simulink model "Assembly"  (R2022b)
settings: Solver=daessc  StartTime=0.0  StopTime=20  MaxStep=1e-3  RelTol=1e-3  AbsTol=1e-3
PreLoadFcn:
  | load environment.mat;
values from neighbouring files (symbols this model uses):
  K_dqdp = 1000    [allData.mat]
  robot =     [allData.mat]
  smoother_length = 4    [allData.mat]
  ts = 0.01    [allData.mat]
undefined symbols (not defined in the file or in its folder): X, Y, Z
libraries: sm_lib x37, nesl_utility x26, dspfactors x8, robotmaniplib x8, simulink x1, dspinverses x1
(part 2 of 2)

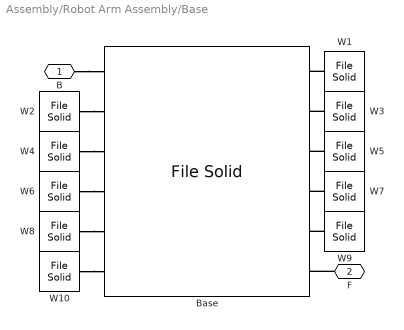
== system Assembly/Robot Arm Assembly/Base ==
  Base : sm_lib/Body Elements/File Solid  ExtGeomFileName=Base.step  UnitType=FromFile  ExtGeomFileUnits=m  StepReaderType=HEX  ExportConvexHullGeometry=off  InertiaType=CalculateFromGeometry  Mass=robot.Solid(19).mass  MassUnits=kg  CenterOfMass=robot.Solid(19).CoM  CenterOfMassUnits=mm  MomentsOfInertia=robot.Solid(19).MoI  MomentsOfInertiaUnits=kg*mm^2  ProductsOfInertia=robot.Solid(19).PoI  ProductsOfInertiaUnits=kg*mm^2  BasedOnType=Density  Density=1000  DensityUnits=kg/m^3  DoExposeReferenceFrame=off  SerializedFrames=<Frames><Frame><Id>Frame1</Id><Value><Name>Origin</Name><Origin><Source>GeometricFeature</Source><FeatureName>segment 442</FeatureName></Origin><PrimaryAxis><DefinedDirection>+Z</DefinedDirection><Source>ReferenceFrame</Source><SourceDirection>-X</SourceDirection><FeatureName></FeatureName></PrimaryAxis><SecondaryAxis><DefinedDirection>+Y</DefinedDirection><Source>ReferenceFrame</Source><SourceDirection>-Y</SourceDirection><FeatureName></FeatureName></SecondaryAxis></Value></Frame><Frame><Id>Frame2</Id><Value><Name>W1</Name><Origin><Source>GeometricFeature</Source><FeatureName>circular curve 177</FeatureName></Origin><PrimaryAxis><DefinedDirection>+Z</DefinedDirection><Source>ReferenceFrame</Source><SourceDirection>+Z</SourceDirection><FeatureName></FeatureName></PrimaryAxis><SecondaryAxis><DefinedDirection>+X</DefinedDirection><Source>ReferenceFrame</Source><SourceDirection>+X</SourceDirection><FeatureName></FeatureName></SecondaryAxis></Value></Frame><Frame><Id>Frame3</Id><Value><Name>W2</Name><Origin><Source>GeometricFeature</Source><FeatureName>circular curve 171</FeatureName></Origin><PrimaryAxis><DefinedDirection>+Z</DefinedDirection><Source>ReferenceFrame</Source><SourceDirection>+Z</SourceDirection><FeatureName></FeatureName></PrimaryAxis><SecondaryAxis><DefinedDirection>+X</DefinedDirection><Source>ReferenceFrame</Source><SourceDirection>+X</SourceDirection><FeatureName></FeatureName></SecondaryAxis></Value></Frame><Frame><Id>Frame4</Id><Value><Name>W3</Name><Origin><Source>GeometricFeature</Source><FeatureName>circular curve 168</FeatureName></Origin><PrimaryAxis><DefinedDirection>+Z</DefinedDirection><Source>ReferenceFrame</Source><SourceDirection>+Z</SourceDirection><FeatureName></FeatureName></PrimaryAxis><SecondaryAxis><DefinedDirection>+X</DefinedDirection><Source>ReferenceFrame</Source><SourceDirection>+X</SourceDirection><FeatureName></FeatureName></SecondaryAxis></Value></Frame><Frame><Id>Frame5</Id><Value><Name>W4</Name><Origin><Source>GeometricFeature</Source><FeatureName>circular curve 174</FeatureName></Origin><PrimaryAxis><DefinedDirection>+Z</DefinedDirection><Source>ReferenceFrame</Source><SourceDirection>+Z</SourceDirection><FeatureName></FeatureName></PrimaryAxis><SecondaryAxis><DefinedDirection>+X</DefinedDirection><Source>ReferenceFrame</Source><SourceDirection>+X</SourceDirection><FeatureName></FeatureName></SecondaryAxis></Value></Frame><Frame><Id>Frame6</Id><Value><Name>W5</Name><Origin><Source>GeometricFeature</Source><FeatureName>circular curve 179</FeatureName></Origin><PrimaryAxis><DefinedDirection>+Z</DefinedDirection><Source>ReferenceFrame</Source><SourceDirection>+Z</SourceDirection><FeatureName></FeatureName></PrimaryAxis><SecondaryAxis><DefinedDirection>+X</DefinedDirection><Source>ReferenceFrame</Source><SourceDirection>+X</SourceDirection><FeatureName></FeatureName></SecondaryAxis></Value></Frame><Frame><Id>Frame7</Id><Value><Name>W6</Name><Origin><Source>GeometricFeature</Source><FeatureName>circular curve 165</FeatureName></Origin><PrimaryAxis><DefinedDirection>+Z</DefinedDirection><Source>ReferenceFrame</Source><SourceDirection>+Z</SourceDirection><FeatureName></FeatureName></PrimaryAxis><SecondaryAxis><DefinedDirection>+X</DefinedDirection><Source>ReferenceFrame</Source><SourceDirection>+X</SourceDirection><FeatureName></FeatureName></SecondaryAxis></Value></Frame><Frame><Id>Frame8</Id><Value><Name>W7</Name><Origin><Source>GeometricFeature</Source><FeatureName>circular curve 157</FeatureName></Origin><PrimaryAxis><DefinedDirection>+Z</DefinedDirection><Source>ReferenceFrame</Source><SourceDirection>+Z</SourceDirection><FeatureName></FeatureName></PrimaryAxis><SecondaryAxis><DefinedDirection>+X</DefinedDirection><Source>ReferenceFrame</Source><SourceDirection>+X</SourceDirection><FeatureName></FeatureName></SecondaryAxis></Value></Frame><Frame><Id>Frame9</Id><Value><Name>W8</Name><Origin><Source>GeometricFeature</Source><FeatureName>circular curve 149</FeatureName></Origin><PrimaryAxis><DefinedDirection>+Z</DefinedDirection><Source>ReferenceFrame</Source><SourceDirection>+Z</SourceDirection><FeatureName></FeatureName></PrimaryAxis><SecondaryAxis><DefinedDirection>+X</DefinedDirection><Source>ReferenceFrame</Source><SourceDirection>+X</SourceDirection><FeatureName></FeatureName></SecondaryAxis></Value></Frame><Frame><Id>Frame10</Id><Value><Name>W9</Name><Origin><Source>GeometricFeature</Source><FeatureName>circular curve 153</FeatureName></Origin><PrimaryAxis><DefinedDirection>+Z</DefinedDirection><Source>ReferenceFrame</Source><SourceDirection>+Z</SourceDirection><FeatureName></FeatureName></PrimaryAxis><SecondaryAxis><DefinedDirection>+X</DefinedDirection><Source>ReferenceFrame</Source><SourceDirection>+X</SourceDirection><FeatureName></FeatureName></SecondaryAxis></Value></Frame><Frame><Id>Frame11</Id><Value><Name>W10</Name><Origin><Source>GeometricFeature</Source><FeatureName>circular curve 161</FeatureName></Origin><PrimaryAxis><DefinedDirection>+Z</DefinedDirection><Source>ReferenceFrame</Source><SourceDirection>+Z</SourceDirection><FeatureName></FeatureName></PrimaryAxis><SecondaryAxis><DefinedDirection>+X</DefinedDirection><Source>ReferenceFrame</Source><SourceDirection>+X</SourceDirection><FeatureName></FeatureName></SecondaryAxis></Value></Frame><Frame><Id>Frame12</Id><Value><Name>F</Name><Origin><Source>GeometricFeature</Source><FeatureName>planar surface 2</FeatureName></Origin><PrimaryAxis><DefinedDirection>+Z</DefinedDirection><Source>ReferenceFrame</Source><SourceDirection>+Z</SourceDirection><FeatureName></FeatureName></PrimaryAxis><SecondaryAxis><DefinedDirection>+X</DefinedDirection><Source>ReferenceFrame</Source><SourceDirection>+X</SourceDirection><FeatureName></FeatureName></SecondaryAxis></Value></Frame></Frames>  GraphicType=FromGeometry  MarkerShape=Sphere  MarkerSize=10  GraphicVisPropType=SimpleVisualProperties  GraphicDiffuseColor=robot.base.color  GraphicSpecularColor=[0.5 0.5 0.5 1.0]  GraphicAmbientColor=[0.15 0.15 0.15 1.0]  GraphicEmissiveColor=[0.0 0.0 0.0 1.0]  GraphicShininess=75  GraphicOpacity=1
  W{1..5} (5 alike) : sm_lib/Body Elements/File Solid  ExtGeomFileName=Wheel.step  UnitType=FromFile  ExtGeomFileUnits=m  StepReaderType=HEX  ExportConvexHullGeometry=off  InertiaType=CalculateFromGeometry  Mass=robot.Solid(1).mass  MassUnits=kg  CenterOfMass=robot.Solid(1).CoM  CenterOfMassUnits=mm  MomentsOfInertia=robot.Solid(1).MoI  MomentsOfInertiaUnits=kg*mm^2  ProductsOfInertia=robot.Solid(1).PoI  ProductsOfInertiaUnits=kg*mm^2  BasedOnType=Density  Density=1000  DensityUnits=kg/m^3  DoExposeReferenceFrame=off  SerializedFrames=<Frames><Frame><Id>Frame1</Id><Value><Name>Wh</Name><Origin><Source>GeometricFeature</Source><FeatureName>circular curve 3</FeatureName></Origin><PrimaryAxis><DefinedDirection>+Z</DefinedDirection><Source>ReferenceFrame</Source><SourceDirection>+Z</SourceDirection><FeatureName></FeatureName></PrimaryAxis><SecondaryAxis><DefinedDirection>+X</DefinedDirection><Source>ReferenceFrame</Source><SourceDirection>+X</SourceDirection><FeatureName></FeatureName></SecondaryAxis></Value></Frame></Frames>  GraphicType=FromGeometry  MarkerShape=Sphere  MarkerSize=10  GraphicVisPropType=SimpleVisualProperties  GraphicDiffuseColor=robot.wheel.color  GraphicSpecularColor=[0.5 0.5 0.5 1.0]  GraphicAmbientColor=[0.15 0.15 0.15 1.0]  GraphicEmissiveColor=[0.0 0.0 0.0 1.0]  GraphicShininess=75  GraphicOpacity=1
  W{6..10} (5 alike) : sm_lib/Body Elements/File Solid  ExtGeomFileName=Wheel.step  UnitType=FromFile  ExtGeomFileUnits=m  StepReaderType=HEX  ExportConvexHullGeometry=off  InertiaType=CalculateFromGeometry  Mass=robot.Solid(1).mass  MassUnits=kg  CenterOfMass=robot.Solid(1).CoM  CenterOfMassUnits=mm  MomentsOfInertia=robot.Solid(1).MoI  MomentsOfInertiaUnits=kg*mm^2  ProductsOfInertia=robot.Solid(1).PoI  ProductsOfInertiaUnits=kg*mm^2  BasedOnType=Density  Density=1000  DensityUnits=kg/m^3  DoExposeReferenceFrame=off  SerializedFrames=<Frames><Frame><Id>Frame1</Id><Value><Name>Wh</Name><Origin><Source>GeometricFeature</Source><FeatureName>circular curve 1</FeatureName></Origin><PrimaryAxis><DefinedDirection>+Z</DefinedDirection><Source>ReferenceFrame</Source><SourceDirection>+Z</SourceDirection><FeatureName></FeatureName></PrimaryAxis><SecondaryAxis><DefinedDirection>+X</DefinedDirection><Source>ReferenceFrame</Source><SourceDirection>+X</SourceDirection><FeatureName></FeatureName></SecondaryAxis></Value></Frame></Frames>  GraphicType=FromGeometry  MarkerShape=Sphere  MarkerSize=10  GraphicVisPropType=SimpleVisualProperties  GraphicDiffuseColor=robot.wheel.color  GraphicSpecularColor=[0.5 0.5 0.5 1.0]  GraphicAmbientColor=[0.15 0.15 0.15 1.0]  GraphicEmissiveColor=[0.0 0.0 0.0 1.0]  GraphicShininess=75  GraphicOpacity=1
  B : PMIOPort  Side=Left
  F : PMIOPort  Port=2  Side=Right
  connections:
  W6/LConn1 -- Base/LConn4
  W4/LConn1 -- Base/LConn3
  W9/LConn1 -- Base/RConn5
  B/RConn1 -- Base/LConn1
  W8/LConn1 -- Base/LConn5
  W1/LConn1 -- Base/RConn1
  W3/LConn1 -- Base/RConn2
  F/RConn1 -- Base/RConn6
  W5/LConn1 -- Base/RConn3
  W10/LConn1 -- Base/LConn6
  W7/LConn1 -- Base/RConn4
  W2/LConn1 -- Base/LConn2

== system Assembly/Robot Arm Assembly/Base2 ==
  Brick Solid : sm_lib/Body Elements/Brick Solid  GraphicAmbientColor=[0.15 0.15 0.15 1.0]  BasedOnType=Density  BrickDimensions=[1 1 1]*0.1  BrickDimensionUnits=m  CenterOfMass=[0 0 0]  CenterOfMassUnits=m  GraphicDiffuseColor=[0.5 0.5 0.5]  Density=1000  DensityUnits=kg/m^3  DoExposeReferenceFrame=on  GraphicEmissiveColor=[0.0 0.0 0.0 1.0]  ExportEntireGeometry=off  SerializedFrames=<Frames/>  MarkerShape=Sphere  MarkerSize=10  GraphicType=FromGeometry  InertiaType=CalculateFromGeometry  Mass=1  MassUnits=kg  MomentsOfInertia=[1 1 1]  MomentsOfInertiaUnits=kg*m^2  GraphicOpacity=1.0  ProductsOfInertia=[0 0 0]  ProductsOfInertiaUnits=kg*m^2  GraphicShininess=75  GraphicSpecularColor=[0.5 0.5 0.5 1.0]  GraphicVisPropType=SimpleVisualProperties
  Rigid Transform : sm_lib/Frames and Transforms/Rigid Transform  TranslationMethod=None  TranslationStandardOffset=0  TranslationLengthUnit=m  TranslationStandardAxis=+Z  TranslationCartesianOffset=[0 0 0]  TranslationROffset=0  TranslationROffsetUnits=m  TranslationZOffset=0  TranslationZOffsetUnits=m  TranslationThetaOffset=0  TranslationThetaOffsetUnits=deg  RotationMethod=AlignedAxes  RotationAngleUnits=deg  RotationStandardAxis=+Z  RotationAngle=0.0  RotationArbitraryAxis=[0 0 1]  FollAlignAxisA=+X  BaseAlignAxisA=-X  FollAlignAxisB=+Y  BaseAlignAxisB=+Z  RotationSequenceAxes=FollowerAxes  RotationSequence=XYX  RotationSequenceAngles=[0 0 0]  RotationSequenceAnglesUnits=deg  RotationMatrix=[1 0 0; 0 1 0; 0 0 1]  Quaternion=[1 0 0 0]
  B : PMIOPort  Side=Left
  F : PMIOPort  Port=2  Side=Right
  connections:
  B/RConn1 -- Brick Solid/RConn1 -- Rigid Transform/LConn1
  Rigid Transform/RConn1 -- F/RConn1

== system Assembly/Robot Arm Assembly/Gripper ==
  Gripper Head : Subsystem
      mask Display: image('GripperHead.png')
  B : PMIOPort  Side=Left
  Ball : PMIOPort  Port=2  Side=Right
  connections:
  B/RConn1 -- Gripper Head/LConn1
  Gripper Head/RConn1 -- Ball/RConn1

== system Assembly/Robot Arm Assembly/Rail ==
  Rail : sm_lib/Body Elements/File Solid  ExtGeomFileName=Rail.step  UnitType=FromFile  ExtGeomFileUnits=m  StepReaderType=HEX  ExportConvexHullGeometry=off  InertiaType=CalculateFromGeometry  Mass=robot.Solid(4).mass  MassUnits=kg  CenterOfMass=robot.Solid(4).CoM  CenterOfMassUnits=mm  MomentsOfInertia=robot.Solid(4).MoI  MomentsOfInertiaUnits=kg*mm^2  ProductsOfInertia=robot.Solid(4).PoI  ProductsOfInertiaUnits=kg*mm^2  BasedOnType=Density  Density=1000  DensityUnits=kg/m^3  DoExposeReferenceFrame=off  SerializedFrames=<Frames><Frame><Id>Frame1</Id><Value><Name>Origin</Name><Origin><Source>GeometricFeature</Source><FeatureName>planar surface 22</FeatureName></Origin><PrimaryAxis><DefinedDirection>+Z</DefinedDirection><Source>ReferenceFrame</Source><SourceDirection>+Z</SourceDirection><FeatureName></FeatureName></PrimaryAxis><SecondaryAxis><DefinedDirection>+X</DefinedDirection><Source>ReferenceFrame</Source><SourceDirection>+X</SourceDirection><FeatureName></FeatureName></SecondaryAxis></Value></Frame><Frame><Id>Frame2</Id><Value><Name>Top</Name><Origin><Source>GeometricFeature</Source><FeatureName>segment 43</FeatureName></Origin><PrimaryAxis><DefinedDirection>+Z</DefinedDirection><Source>ReferenceFrame</Source><SourceDirection>+X</SourceDirection><FeatureName></FeatureName></PrimaryAxis><SecondaryAxis><DefinedDirection>+Y</DefinedDirection><Source>ReferenceFrame</Source><SourceDirection>+Y</SourceDirection><FeatureName></FeatureName></SecondaryAxis></Value></Frame></Frames>  GraphicType=FromGeometry  MarkerShape=Sphere  MarkerSize=10  GraphicVisPropType=SimpleVisualProperties  GraphicDiffuseColor=robot.rail.color  GraphicSpecularColor=[0.5 0.5 0.5 1.0]  GraphicAmbientColor=[0.15 0.15 0.15 1.0]  GraphicEmissiveColor=[0.0 0.0 0.0 1.0]  GraphicShininess=75  GraphicOpacity=1
  B : PMIOPort  Side=Left
  F : PMIOPort  Port=2  Side=Right
  connections:
  F/RConn1 -- Rail/RConn1
  Rail/LConn1 -- B/RConn1

== system Assembly/Robot Arm Assembly/Wrist ==
  Wrist : sm_lib/Body Elements/File Solid  ExtGeomFileName=Wrist.step  UnitType=FromFile  ExtGeomFileUnits=m  StepReaderType=HEX  ExportConvexHullGeometry=off  InertiaType=CalculateFromGeometry  Mass=robot.Solid(9).mass  MassUnits=kg  CenterOfMass=robot.Solid(9).CoM  CenterOfMassUnits=mm  MomentsOfInertia=robot.Solid(9).MoI  MomentsOfInertiaUnits=kg*mm^2  ProductsOfInertia=robot.Solid(9).PoI  ProductsOfInertiaUnits=kg*mm^2  BasedOnType=Density  Density=1000  DensityUnits=kg/m^3  DoExposeReferenceFrame=off  SerializedFrames=<Frames><Frame><Id>Frame1</Id><Value><Name>B</Name><Origin><Source>GeometricFeature</Source><FeatureName>planar surface 1</FeatureName></Origin><PrimaryAxis><DefinedDirection>+Z</DefinedDirection><Source>ReferenceFrame</Source><SourceDirection>+X</SourceDirection><FeatureName></FeatureName></PrimaryAxis><SecondaryAxis><DefinedDirection>+Y</DefinedDirection><Source>ReferenceFrame</Source><SourceDirection>+Y</SourceDirection><FeatureName></FeatureName></SecondaryAxis></Value></Frame><Frame><Id>Frame2</Id><Value><Name>F</Name><Origin><Source>GeometricFeature</Source><FeatureName>planar surface 14</FeatureName></Origin><PrimaryAxis><DefinedDirection>+Z</DefinedDirection><Source>ReferenceFrame</Source><SourceDirection>+Z</SourceDirection><FeatureName></FeatureName></PrimaryAxis><SecondaryAxis><DefinedDirection>+X</DefinedDirection><Source>ReferenceFrame</Source><SourceDirection>+X</SourceDirection><FeatureName></FeatureName></SecondaryAxis></Value></Frame></Frames>  GraphicType=FromGeometry  MarkerShape=Sphere  MarkerSize=10  GraphicVisPropType=SimpleVisualProperties  GraphicDiffuseColor=robot.wrist.color  GraphicSpecularColor=[0.5 0.5 0.5 1.0]  GraphicAmbientColor=[0.15 0.15 0.15 1.0]  GraphicEmissiveColor=[0.0 0.0 0.0 1.0]  GraphicShininess=75  GraphicOpacity=1
  B : PMIOPort  Side=Left
  F : PMIOPort  Port=2  Side=Right
  connections:
  Wrist/LConn1 -- B/RConn1
  F/RConn1 -- Wrist/RConn1

== system Assembly/Self Motion/CondNum ==
  J : Inport
  Product2 : Product  Inputs=*  SaturateOnIntegerOverflow=on  OutDataTypeStr=Inherit: Same as first input
  Singular Value Decomposition : dspfactors/Singular Value Decomposition  wantv=on  wanterr=off  SimulateUsing=Interpreted execution
  Terminator : Terminator
  Terminator1 : Terminator
  p : Outport
  wires:
  Product2/1 -> p/1
  Singular Value Decomposition/2 -> Product2/1
  Singular Value Decomposition/1 -> Terminator1/1
  J/1 -> Singular Value Decomposition/1
  Singular Value Decomposition/3 -> Terminator/1

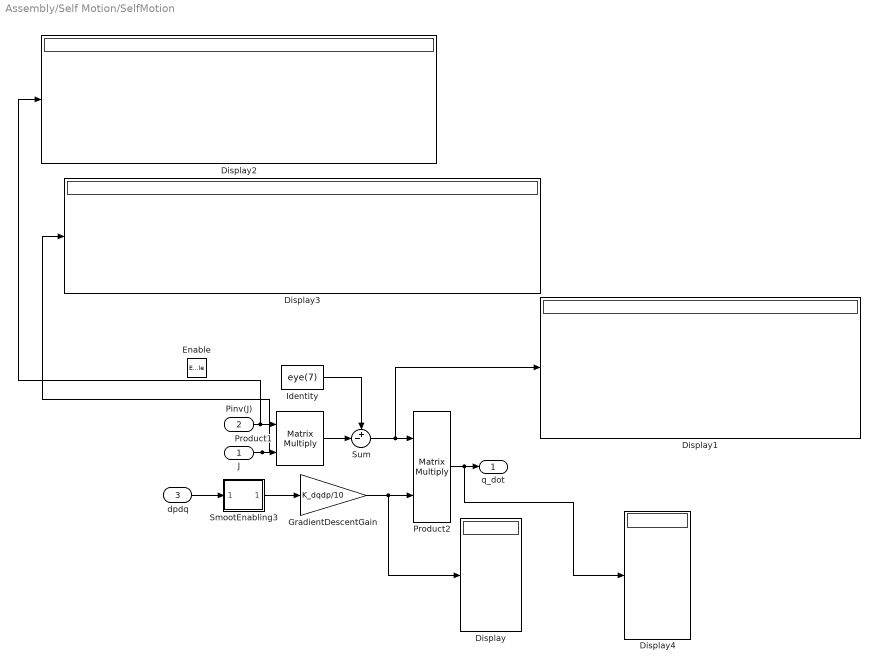
== system Assembly/Self Motion/SelfMotion ==
  J : Inport
  Pinv(J) : Inport  Port=2
  dpdq : Inport  Port=3
  Enable : EnablePort  StatesWhenEnabling=reset
  Display{,1..4} (5 alike) : Display
  GradientDescentGain : Gain  Gain=K_dqdp/10  SaturateOnIntegerOverflow=on  OutDataTypeStr=Inherit: Same as input  ParamDataTypeStr=Inherit: Same as input
  Identity : Constant  Value=eye(7)
  Product1 : Product  Inputs=**  Multiplication=Matrix(*)  SaturateOnIntegerOverflow=on  OutDataTypeStr=Inherit: Same as first input
  Product2 : Product  Inputs=**  Multiplication=Matrix(*)  SaturateOnIntegerOverflow=on  OutDataTypeStr=Inherit: Same as first input
  SmootEnabling3 : Subsystem  TreatAsAtomicUnit=on
  Sum : Sum  Inputs=+-|  SaturateOnIntegerOverflow=on
  q_dot : Outport
  wires:
  GradientDescentGain/1 -> Display/1, Product2/2
  Product2/1 -> Display4/1, q_dot/1
  J/1 -> Display3/1, Product1/2
  Pinv(J)/1 -> Display2/1, Product1/1
  dpdq/1 -> SmootEnabling3/1(In1)
  Product1/1 -> Sum/2
  Sum/1 -> Display1/1, Product2/1
  Identity/1 -> Sum/1
  SmootEnabling3/1(Out1) -> GradientDescentGain/1

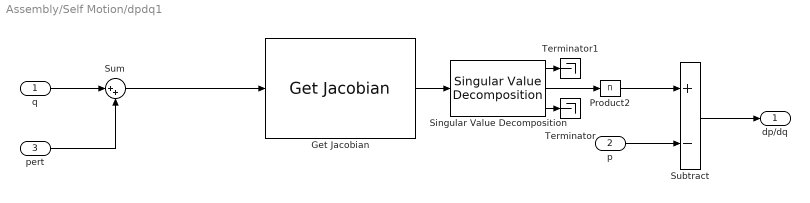
== system Assembly/Self Motion/dpdq1 ==
  q : Inport
  p : Inport  Port=2
  pert : Inport  Port=3
  Get Jacobian : robotmaniplib/Get Jacobian  RigidBodyTree=robotTree  EndEffector=Body7  SimulateUsing=Interpreted execution
  Product2 : Product  Inputs=*  SaturateOnIntegerOverflow=on  OutDataTypeStr=Inherit: Same as first input
  Singular Value Decomposition : dspfactors/Singular Value Decomposition  wantv=on  wanterr=off  SimulateUsing=Interpreted execution
  Subtract : Sum  Inputs=+-
  Sum : Sum  Inputs=|++
  Terminator : Terminator
  Terminator1 : Terminator
  dp/dq : Outport
  wires:
  Singular Value Decomposition/2 -> Product2/1
  Product2/1 -> Subtract/1
  Get Jacobian/1 -> Singular Value Decomposition/1
  q/1 -> Sum/1
  Sum/1 -> Get Jacobian/1
  p/1 -> Subtract/2
  Subtract/1 -> dp/dq/1
  Singular Value Decomposition/3 -> Terminator/1
  Singular Value Decomposition/1 -> Terminator1/1
  pert/1 -> Sum/2

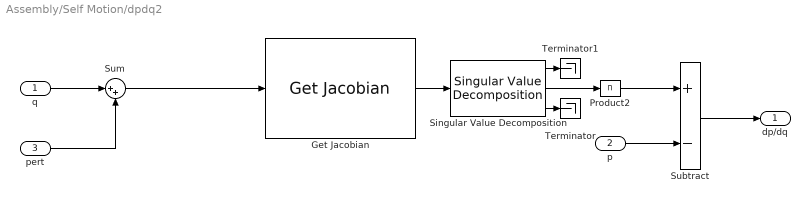
== system Assembly/Self Motion/dpdq2 ==
  q : Inport
  p : Inport  Port=2
  pert : Inport  Port=3
  Get Jacobian : robotmaniplib/Get Jacobian  RigidBodyTree=robotTree  EndEffector=Body7  SimulateUsing=Interpreted execution
  Product2 : Product  Inputs=*  SaturateOnIntegerOverflow=on  OutDataTypeStr=Inherit: Same as first input
  Singular Value Decomposition : dspfactors/Singular Value Decomposition  wantv=on  wanterr=off  SimulateUsing=Interpreted execution
  Subtract : Sum  Inputs=+-
  Sum : Sum  Inputs=|++
  Terminator : Terminator
  Terminator1 : Terminator
  dp/dq : Outport
  wires:
  pert/1 -> Sum/2
  Singular Value Decomposition/1 -> Terminator1/1
  Singular Value Decomposition/3 -> Terminator/1
  Subtract/1 -> dp/dq/1
  p/1 -> Subtract/2
  Sum/1 -> Get Jacobian/1
  q/1 -> Sum/1
  Get Jacobian/1 -> Singular Value Decomposition/1
  Product2/1 -> Subtract/1
  Singular Value Decomposition/2 -> Product2/1

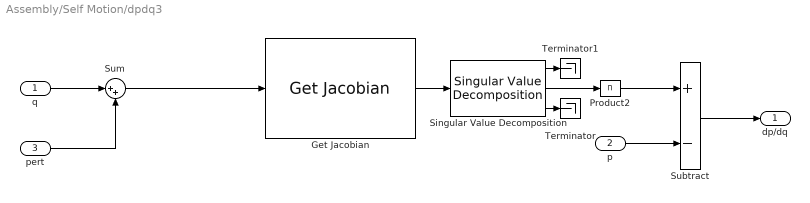
== system Assembly/Self Motion/dpdq3 ==
  q : Inport
  p : Inport  Port=2
  pert : Inport  Port=3
  Get Jacobian : robotmaniplib/Get Jacobian  RigidBodyTree=robotTree  EndEffector=Body7  SimulateUsing=Interpreted execution
  Product2 : Product  Inputs=*  SaturateOnIntegerOverflow=on  OutDataTypeStr=Inherit: Same as first input
  Singular Value Decomposition : dspfactors/Singular Value Decomposition  wantv=on  wanterr=off  SimulateUsing=Interpreted execution
  Subtract : Sum  Inputs=+-
  Sum : Sum  Inputs=|++
  Terminator : Terminator
  Terminator1 : Terminator
  dp/dq : Outport
  wires:
  Singular Value Decomposition/2 -> Product2/1
  Product2/1 -> Subtract/1
  Get Jacobian/1 -> Singular Value Decomposition/1
  q/1 -> Sum/1
  Sum/1 -> Get Jacobian/1
  p/1 -> Subtract/2
  Subtract/1 -> dp/dq/1
  Singular Value Decomposition/3 -> Terminator/1
  Singular Value Decomposition/1 -> Terminator1/1
  pert/1 -> Sum/2

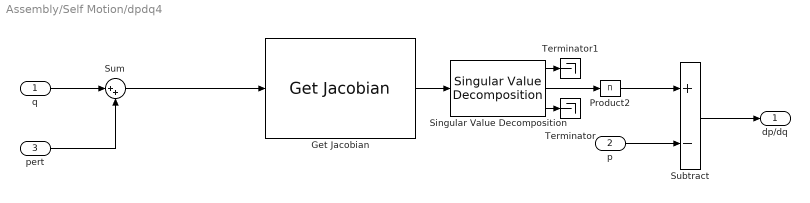
== system Assembly/Self Motion/dpdq4 ==
  q : Inport
  p : Inport  Port=2
  pert : Inport  Port=3
  Get Jacobian : robotmaniplib/Get Jacobian  RigidBodyTree=robotTree  EndEffector=Body7  SimulateUsing=Interpreted execution
  Product2 : Product  Inputs=*  SaturateOnIntegerOverflow=on  OutDataTypeStr=Inherit: Same as first input
  Singular Value Decomposition : dspfactors/Singular Value Decomposition  wantv=on  wanterr=off  SimulateUsing=Interpreted execution
  Subtract : Sum  Inputs=+-
  Sum : Sum  Inputs=|++
  Terminator : Terminator
  Terminator1 : Terminator
  dp/dq : Outport
  wires:
  pert/1 -> Sum/2
  Singular Value Decomposition/1 -> Terminator1/1
  Singular Value Decomposition/3 -> Terminator/1
  Subtract/1 -> dp/dq/1
  p/1 -> Subtract/2
  Sum/1 -> Get Jacobian/1
  q/1 -> Sum/1
  Get Jacobian/1 -> Singular Value Decomposition/1
  Product2/1 -> Subtract/1
  Singular Value Decomposition/2 -> Product2/1

== system Assembly/Self Motion/dpdq5 ==
  q : Inport
  p : Inport  Port=2
  pert : Inport  Port=3
  Get Jacobian : robotmaniplib/Get Jacobian  RigidBodyTree=robotTree  EndEffector=Body7  SimulateUsing=Interpreted execution
  Product2 : Product  Inputs=*  SaturateOnIntegerOverflow=on  OutDataTypeStr=Inherit: Same as first input
  Singular Value Decomposition : dspfactors/Singular Value Decomposition  wantv=on  wanterr=off  SimulateUsing=Interpreted execution
  Subtract : Sum  Inputs=+-
  Sum : Sum  Inputs=|++
  Terminator : Terminator
  Terminator1 : Terminator
  dp/dq : Outport
  wires:
  Singular Value Decomposition/2 -> Product2/1
  Product2/1 -> Subtract/1
  Get Jacobian/1 -> Singular Value Decomposition/1
  q/1 -> Sum/1
  Sum/1 -> Get Jacobian/1
  p/1 -> Subtract/2
  Subtract/1 -> dp/dq/1
  Singular Value Decomposition/3 -> Terminator/1
  Singular Value Decomposition/1 -> Terminator1/1
  pert/1 -> Sum/2

== system Assembly/Self Motion/dpdq6 ==
  q : Inport
  p : Inport  Port=2
  pert : Inport  Port=3
  Get Jacobian : robotmaniplib/Get Jacobian  RigidBodyTree=robotTree  EndEffector=Body7  SimulateUsing=Interpreted execution
  Product2 : Product  Inputs=*  SaturateOnIntegerOverflow=on  OutDataTypeStr=Inherit: Same as first input
  Singular Value Decomposition : dspfactors/Singular Value Decomposition  wantv=on  wanterr=off  SimulateUsing=Interpreted execution
  Subtract : Sum  Inputs=+-
  Sum : Sum  Inputs=|++
  Terminator : Terminator
  Terminator1 : Terminator
  dp/dq : Outport
  wires:
  pert/1 -> Sum/2
  Singular Value Decomposition/1 -> Terminator1/1
  Singular Value Decomposition/3 -> Terminator/1
  Subtract/1 -> dp/dq/1
  p/1 -> Subtract/2
  Sum/1 -> Get Jacobian/1
  q/1 -> Sum/1
  Get Jacobian/1 -> Singular Value Decomposition/1
  Product2/1 -> Subtract/1
  Singular Value Decomposition/2 -> Product2/1

== system Assembly/Self Motion/dpdq7 ==
  q : Inport
  p : Inport  Port=2
  pert : Inport  Port=3
  Get Jacobian : robotmaniplib/Get Jacobian  RigidBodyTree=robotTree  EndEffector=Body7  SimulateUsing=Interpreted execution
  Product2 : Product  Inputs=*  SaturateOnIntegerOverflow=on  OutDataTypeStr=Inherit: Same as first input
  Singular Value Decomposition : dspfactors/Singular Value Decomposition  wantv=on  wanterr=off  SimulateUsing=Interpreted execution
  Subtract : Sum  Inputs=+-
  Sum : Sum  Inputs=|++
  Terminator : Terminator
  Terminator1 : Terminator
  dp/dq : Outport
  wires:
  Singular Value Decomposition/2 -> Product2/1
  Product2/1 -> Subtract/1
  Get Jacobian/1 -> Singular Value Decomposition/1
  q/1 -> Sum/1
  Sum/1 -> Get Jacobian/1
  p/1 -> Subtract/2
  Subtract/1 -> dp/dq/1
  Singular Value Decomposition/3 -> Terminator/1
  Singular Value Decomposition/1 -> Terminator1/1
  pert/1 -> Sum/2

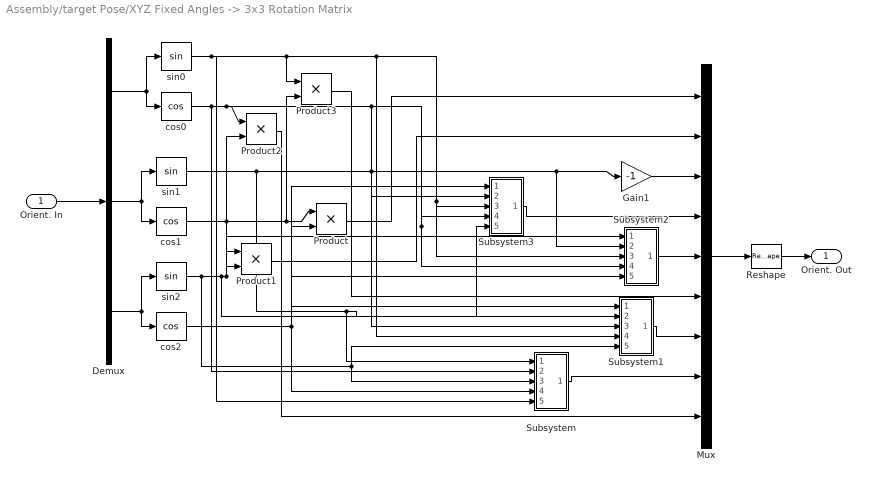
== system Assembly/target Pose/XYZ Fixed Angles -> 3x3 Rotation Matrix ==
  Orient. In : Inport
  Demux : Demux  Outputs=3
      settings: DisplayOption=none
  Gain1 : Gain  Gain=-1  SaturateOnIntegerOverflow=on  OutDataTypeStr=Inherit: Same as input  ParamDataTypeStr=Inherit: Same as input
  Mux : Mux  Inputs=9
  Product{,1..3} (4 alike) : Product  InputSameDT=on  SaturateOnIntegerOverflow=on  OutDataTypeStr=Inherit: Same as first input
  Reshape : Reshape  OutputDimensionality=Customize  OutputDimensions=[3,3]
  Subsystem : Subsystem
  Subsystem1 : Subsystem
  Subsystem2 : Subsystem
  Subsystem3 : Subsystem
  cos0 : Trigonometry  Operator=cos
  cos1 : Trigonometry  Operator=cos
  cos2 : Trigonometry  Operator=cos
  sin0 : Trigonometry
  sin1 : Trigonometry
  sin2 : Trigonometry
  Orient. Out : Outport
  wires:
  Demux/3 -> cos2/1, sin2/1
  Demux/2 -> cos1/1, sin1/1
  Demux/1 -> cos0/1, sin0/1
  Orient. In/1 -> Demux/1
  Mux/1 -> Reshape/1
  sin0/1 -> Subsystem/5(In5), Subsystem1/4(In4), Subsystem3/3(In3), Subsystem2/3(In3), Product3/1
  cos0/1 -> Subsystem/2(In2), Subsystem1/3(In3), Subsystem3/4(In4), Subsystem2/4(In4), Product2/1
  sin2/1 -> Subsystem1/5(In5), Subsystem/3(In3), Subsystem3/5(In5), Subsystem2/1(In1), Product1/2
  sin1/1 -> Subsystem1/2(In2), Subsystem/1(In1), Subsystem3/2(In2), Subsystem2/2(In2), Gain1/1
  cos2/1 -> Subsystem3/1(In1), Subsystem2/5(In5), Subsystem1/1(In1), Subsystem/4(In4), Product/2
  Subsystem/1(Out1) -> Mux/8
  Subsystem3/1(Out1) -> Mux/4
  Subsystem1/1(Out1) -> Mux/7
  Subsystem2/1(Out1) -> Mux/5
  Product3/1 -> Mux/6
  Product2/1 -> Mux/9
  Gain1/1 -> Mux/3
  Product1/1 -> Mux/2
  cos1/1 -> Product3/2, Product/1, Product2/2, Product1/1
  Product/1 -> Mux/1
  Reshape/1 -> Orient. Out/1

== system Assembly/End Effector Motion/6DOF Traj Gen/Cart Pos Error Calc ==
  Desired Position : Inport
  Desired Orientation : Inport  Port=2
  Current Position : Inport  Port=3
  Current Orientation : Inport  Port=4
  "3x3 Rotation Matrix -> Skew Vector" : Subsystem  mask(Orientation Conversion){}
      mask help:
      | Converts from a 3x3 Rotation Matrix orientation representation into the Skew Vector orientation representation. The Skew Vector representation is only valid for small orientation errors.
      |
      | Input: [3 3] rotation matrix R
      | Output: [3 1] skew vector [dx dy dz]
      |
      | where dx, dy ,dz, are small rotation about the x, y and z axes expressed  in radians.
  Mux : Mux  Inputs=2
  R1 * R2^T1 : Subsystem
  Sum1 : Sum  Inputs=+-  SaturateOnIntegerOverflow=on
  Pose Error : Outport
  wires:
  Desired Orientation/1 -> R1 * R2^T1/1(Orient. 1 In)
  Sum1/1 -> Mux/2
  R1 * R2^T1/1(Orient. Out) -> "3x3 Rotation Matrix -> Skew Vector"/1(Orient. In)
  Desired Position/1 -> Sum1/1
  Current Orientation/1 -> R1 * R2^T1/2(Orient. 2 In)
  Current Position/1 -> Sum1/2
  Mux/1 -> Pose Error/1
  "3x3 Rotation Matrix -> Skew Vector"/1(Orient. Out) -> Mux/1

== system Assembly/Robot Arm Assembly/Gripper/Gripper Head ==
  Gripper Head : sm_lib/Body Elements/File Solid  ExtGeomFileName=GripperHead.step  UnitType=FromFile  ExtGeomFileUnits=m  StepReaderType=HEX  ExportConvexHullGeometry=off  InertiaType=CalculateFromGeometry  Mass=robot.Solid(16).mass  MassUnits=kg  CenterOfMass=robot.Solid(16).CoM  CenterOfMassUnits=mm  MomentsOfInertia=robot.Solid(16).MoI  MomentsOfInertiaUnits=kg*mm^2  ProductsOfInertia=robot.Solid(16).PoI  ProductsOfInertiaUnits=kg*mm^2  BasedOnType=Density  Density=1000  DensityUnits=kg/m^3  DoExposeReferenceFrame=off  SerializedFrames=<Frames><Frame><Id>Frame1</Id><Value><Name>B</Name><Origin><Source>GeometricFeature</Source><FeatureName>planar surface 8</FeatureName></Origin><PrimaryAxis><DefinedDirection>+Z</DefinedDirection><Source>ReferenceFrame</Source><SourceDirection>+Z</SourceDirection><FeatureName></FeatureName></PrimaryAxis><SecondaryAxis><DefinedDirection>+X</DefinedDirection><Source>ReferenceFrame</Source><SourceDirection>+X</SourceDirection><FeatureName></FeatureName></SecondaryAxis></Value></Frame><Frame><Id>Frame2</Id><Value><Name>Front</Name><Origin><Source>GeometricFeature</Source><FeatureName>planar surface 36</FeatureName></Origin><PrimaryAxis><DefinedDirection>+Z</DefinedDirection><Source>ReferenceFrame</Source><SourceDirection>-Z</SourceDirection><FeatureName></FeatureName></PrimaryAxis><SecondaryAxis><DefinedDirection>+X</DefinedDirection><Source>ReferenceFrame</Source><SourceDirection>+X</SourceDirection><FeatureName></FeatureName></SecondaryAxis></Value></Frame><Frame><Id>Frame3</Id><Value><Name>Gripper1</Name><Origin><Source>GeometricFeature</Source><FeatureName>circular curve 5</FeatureName></Origin><PrimaryAxis><DefinedDirection>+Z</DefinedDirection><Source>ReferenceFrame</Source><SourceDirection>-Y</SourceDirection><FeatureName></FeatureName></PrimaryAxis><SecondaryAxis><DefinedDirection>+X</DefinedDirection><Source>ReferenceFrame</Source><SourceDirection>+X</SourceDirection><FeatureName></FeatureName></SecondaryAxis></Value></Frame><Frame><Id>Frame4</Id><Value><Name>Gripper2</Name><Origin><Source>GeometricFeature</Source><FeatureName>circular curve 6</FeatureName></Origin><PrimaryAxis><DefinedDirection>+Z</DefinedDirection><Source>ReferenceFrame</Source><SourceDirection>-Y</SourceDirection><FeatureName></FeatureName></PrimaryAxis><SecondaryAxis><DefinedDirection>+X</DefinedDirection><Source>ReferenceFrame</Source><SourceDirection>+X</SourceDirection><FeatureName></FeatureName></SecondaryAxis></Value></Frame></Frames>  GraphicType=FromGeometry  MarkerShape=Sphere  MarkerSize=10  GraphicVisPropType=SimpleVisualProperties  GraphicDiffuseColor=robot.gripper.color  GraphicSpecularColor=[0.5 0.5 0.5 1.0]  GraphicAmbientColor=[0.15 0.15 0.15 1.0]  GraphicEmissiveColor=[0.0 0.0 0.0 1.0]  GraphicShininess=75  GraphicOpacity=1
  Rigid Transform : sm_lib/Frames and Transforms/Rigid Transform  TranslationMethod=Cartesian  TranslationStandardOffset=0  TranslationLengthUnit=m  TranslationStandardAxis=+Z  TranslationCartesianOffset=robot.gripper.offset  TranslationROffset=0  TranslationROffsetUnits=m  TranslationZOffset=0  TranslationZOffsetUnits=m  TranslationThetaOffset=0  TranslationThetaOffsetUnits=deg  RotationMethod=None  RotationAngleUnits=deg  RotationStandardAxis=+Z  RotationAngle=0.0  RotationArbitraryAxis=[0 0 1]  FollAlignAxisA=+X  BaseAlignAxisA=+Y  FollAlignAxisB=+Y  BaseAlignAxisB=+Z  RotationSequenceAxes=FollowerAxes  RotationSequence=XYX  RotationSequenceAngles=[0 0 0]  RotationSequenceAnglesUnits=deg  RotationMatrix=[1 0 0; 0 1 0; 0 0 1]  Quaternion=[1 0 0 0]
  B : PMIOPort  Side=Left
  Ball : PMIOPort  Port=2  Side=Right
  connections:
  Gripper Head/LConn1 -- B/RConn1
  Ball/RConn1 -- Rigid Transform/RConn1
  Rigid Transform/LConn1 -- Gripper Head/RConn1

== system Assembly/Self Motion/SelfMotion/SmootEnabling3 ==
  In1 : Inport
  Constant : Constant  Value=ts/smoother_length
  Product : Product  SaturateOnIntegerOverflow=on  OutDataTypeStr=Inherit: Same as first input
  Saturation : Saturate  UpperLimit=1  LowerLimit=0
  Sum : Sum  Inputs=|++  SaturateOnIntegerOverflow=on
  Unit Delay : UnitDelay  SampleTime=ts
  Out1 : Outport
  wires:
  Constant/1 -> Sum/1
  Unit Delay/1 -> Saturation/1
  Sum/1 -> Unit Delay/1
  Product/1 -> Out1/1
  Saturation/1 -> Sum/2, Product/2
  In1/1 -> Product/1

== system Assembly/target Pose/XYZ Fixed Angles -> 3x3 Rotation Matrix/Subsystem ==
  In1 : Inport
  In2 : Inport  Port=2
  In3 : Inport  Port=3
  In4 : Inport  Port=4
  In5 : Inport  Port=5
  Product10 : Product  Inputs=3  InputSameDT=on  SaturateOnIntegerOverflow=on  OutDataTypeStr=Inherit: Same as first input
  Product11 : Product  InputSameDT=on  SaturateOnIntegerOverflow=on  OutDataTypeStr=Inherit: Same as first input
  Sum3 : Sum  Inputs=+-  InputSameDT=on  SaturateOnIntegerOverflow=on  OutDataTypeStr=Inherit: Same as first input
  Out1 : Outport
  wires:
  Sum3/1 -> Out1/1
  In5/1 -> Product11/2
  In4/1 -> Product11/1
  In2/1 -> Product10/2
  In1/1 -> Product10/1
  In3/1 -> Product10/3
  Product11/1 -> Sum3/2
  Product10/1 -> Sum3/1

== system Assembly/target Pose/XYZ Fixed Angles -> 3x3 Rotation Matrix/Subsystem1 ==
  In1 : Inport
  In2 : Inport  Port=2
  In3 : Inport  Port=3
  In4 : Inport  Port=4
  In5 : Inport  Port=5
  Product6 : Product  Inputs=3  InputSameDT=on  SaturateOnIntegerOverflow=on  OutDataTypeStr=Inherit: Same as first input
  Product7 : Product  InputSameDT=on  SaturateOnIntegerOverflow=on  OutDataTypeStr=Inherit: Same as first input
  Sum1 : Sum  InputSameDT=on  SaturateOnIntegerOverflow=on  OutDataTypeStr=Inherit: Same as first input
  Out1 : Outport
  wires:
  Sum1/1 -> Out1/1
  In2/1 -> Product6/2
  In5/1 -> Product7/2
  In4/1 -> Product7/1
  In3/1 -> Product6/3
  In1/1 -> Product6/1
  Product7/1 -> Sum1/2
  Product6/1 -> Sum1/1

== system Assembly/target Pose/XYZ Fixed Angles -> 3x3 Rotation Matrix/Subsystem2 ==
  In1 : Inport
  In2 : Inport  Port=2
  In3 : Inport  Port=3
  In4 : Inport  Port=4
  In5 : Inport  Port=5
  Product4 : Product  Inputs=3  InputSameDT=on  SaturateOnIntegerOverflow=on  OutDataTypeStr=Inherit: Same as first input
  Product5 : Product  InputSameDT=on  SaturateOnIntegerOverflow=on  OutDataTypeStr=Inherit: Same as first input
  Sum : Sum  InputSameDT=on  SaturateOnIntegerOverflow=on  OutDataTypeStr=Inherit: Same as first input
  Out1 : Outport
  wires:
  Sum/1 -> Out1/1
  In4/1 -> Product5/1
  In5/1 -> Product5/2
  In3/1 -> Product4/3
  In2/1 -> Product4/2
  In1/1 -> Product4/1
  Product5/1 -> Sum/2
  Product4/1 -> Sum/1

== system Assembly/target Pose/XYZ Fixed Angles -> 3x3 Rotation Matrix/Subsystem3 ==
  In1 : Inport
  In2 : Inport  Port=2
  In3 : Inport  Port=3
  In4 : Inport  Port=4
  In5 : Inport  Port=5
  Product8 : Product  Inputs=3  InputSameDT=on  SaturateOnIntegerOverflow=on  OutDataTypeStr=Inherit: Same as first input
  Product9 : Product  InputSameDT=on  SaturateOnIntegerOverflow=on  OutDataTypeStr=Inherit: Same as first input
  Sum2 : Sum  Inputs=+-  InputSameDT=on  SaturateOnIntegerOverflow=on  OutDataTypeStr=Inherit: Same as first input
  Out1 : Outport
  wires:
  Sum2/1 -> Out1/1
  In4/1 -> Product9/1
  In3/1 -> Product8/3
  In5/1 -> Product9/2
  In2/1 -> Product8/2
  In1/1 -> Product8/1
  Product9/1 -> Sum2/2
  Product8/1 -> Sum2/1

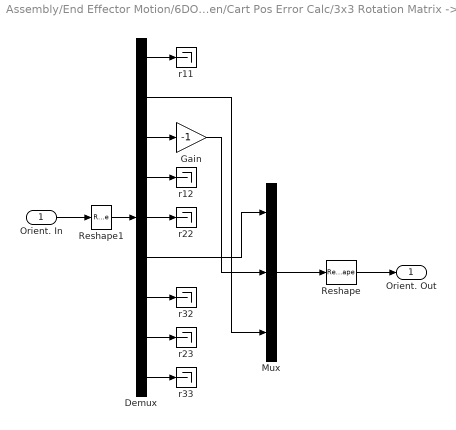
== system Assembly/End Effector Motion/6DOF Traj Gen/Cart Pos Error Calc/3x3 Rotation Matrix -> Skew Vector ==
  Orient. In : Inport
  Demux : Demux  Outputs=9
      settings: DisplayOption=none
  Gain : Gain  Gain=-1  SaturateOnIntegerOverflow=on  OutDataTypeStr=Inherit: Same as input  ParamDataTypeStr=Inherit: Same as input
  Mux : Mux  Inputs=3
  Reshape : Reshape  OutputDimensionality=Column vector (2-D)
  Reshape1 : Reshape
  r{11..12,22..23,32..33} (6 alike) : Terminator
  Orient. Out : Outport
  wires:
  Reshape1/1 -> Demux/1
  Reshape/1 -> Orient. Out/1
  Demux/2 -> Mux/3
  Gain/1 -> Mux/2
  Demux/3 -> Gain/1
  Demux/7 -> r32/1
  Demux/9 -> r33/1
  Demux/8 -> r23/1
  Demux/5 -> r22/1
  Demux/4 -> r12/1
  Demux/1 -> r11/1
  Demux/6 -> Mux/1
  Mux/1 -> Reshape/1
  Orient. In/1 -> Reshape1/1

== system Assembly/End Effector Motion/6DOF Traj Gen/Cart Pos Error Calc/R1 * R2^T1 ==
  Orient. 1 In : Inport
  Orient. 2 In : Inport  Port=2
  Matrix Multiply : Product  Multiplication=Matrix(*)
  Transpose : Math  Operator=transpose
  Orient. Out : Outport  InitialOutput=0
  wires:
  Orient. 2 In/1 -> Transpose/1
  Orient. 1 In/1 -> Matrix Multiply/1
  Transpose/1 -> Matrix Multiply/2
  Matrix Multiply/1 -> Orient. Out/1
